simulink model "MissionSupervisor"  (R2020a)
settings: Solver=VariableStepAuto  StartTime=0.0  StopTime=10.0  RelTol=1e-3
undefined symbols (not defined in the file or in its folder): DiscIntNeverNeededParam
libraries: simulink x2
(part 1 of 2)
settings Model: PauseTimes=1  PacingRate=0.350000  Creator=User  LastModifiedBy=User

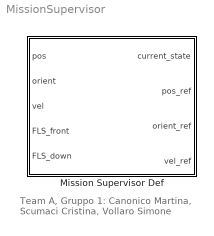
== system MissionSupervisor ==
  note: Team A, Gruppo 1:
      | Canonico Martina, Scumaci Cristina, Vollaro Simone
  Mission Supervisor Def : Subsystem

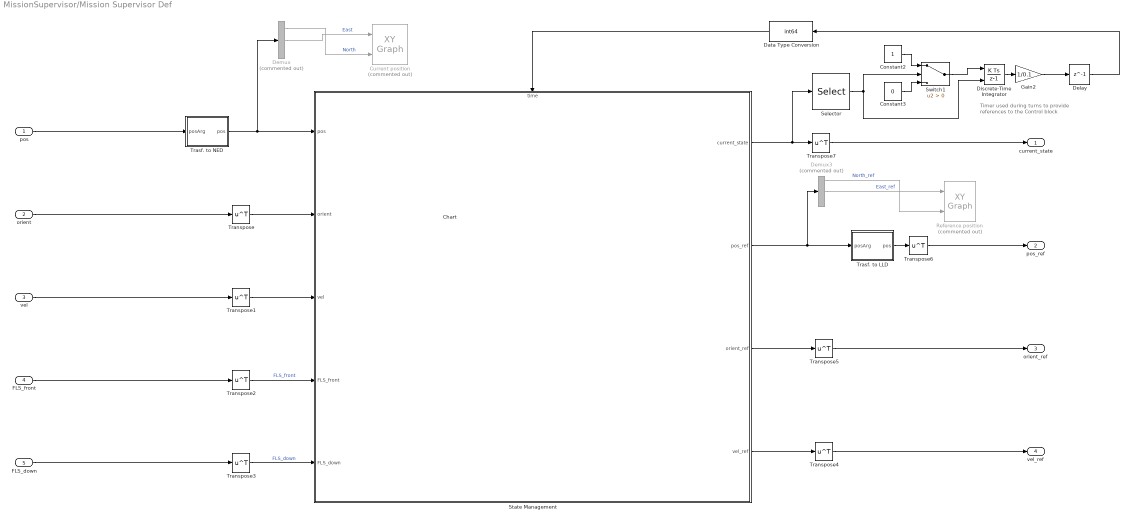
== system MissionSupervisor/Mission Supervisor Def ==
  note: Timer used during turns to
      | provide references to the Control block
  pos : Inport
  orient : Inport  Port=2  PortDimensions=[3 1]
  vel : Inport  Port=3  PortDimensions=[6 1]
  FLS_front : Inport  Port=4  PortDimensions=1
  FLS_down : Inport  Port=5  PortDimensions=1
  Chart : Stateflow chart  TreatAsAtomicUnit=on
  Constant2 : Constant
  Constant3 : Constant  Value=0
  Current position : simulink/Sinks/XY Graph  Commented=on  xmin=0  xmax=150  ymin=0  ymax=150  st=-1
  Data Type Conversion : DataTypeConversion  OutDataTypeStr=int64
  Delay : Delay  DelayLength=1  SampleTime=0.1
  Demux : Demux  Commented=on  Outputs=3
  Demux3 : Demux  Commented=on  Outputs=3
  Discrete-Time Integrator : DiscreteIntegrator  ExternalReset=falling  SampleTime=0.1  ICPrevOutput=DiscIntNeverNeededParam  ICPrevScaledInput=DiscIntNeverNeededParam
  Gain2 : Gain  Gain=1/0.1
  Reference position : simulink/Sinks/XY Graph  Commented=on  xmin=0  xmax=150  ymin=0  ymax=150  st=-1
  Selector : Selector  InputPortWidth=8  IndexOptions=Index vector (dialog)  Indices=4  OutputSizes=1
  State Management : Stateflow chart  TreatAsAtomicUnit=on
      settings: PortSchema="{\"entries\":[{\"content\":{\"sides\":[{\"content\":{\"connectorIds\":[\"In1\",\"In2\",\"In3\",\"In4\",\"In5\"]},\"type\":\"ConnectorPlacement.EquallySpacedRectSide\",\"uuid\":\"b4d768e0-b402-4324-9a12-614211dc6b85\"},{\"content\":{\"connectorIds\":[\"Out1\",\"Out2\",\"Out3\",\"Out4\"],\"side\":\"RIGHT\"},\"type\":\"ConnectorPlacement.EquallySpacedRectSide\",\"uuid\":\"64a4c54a-28a4-456f-aa67-ad7da5d6855f\"},{\"content\":{\"connectorIds\":[\"In6\"],\"side\":\"TOP\"},\"type\":\"ConnectorPlacement.EquallySpacedRectSide\",\"uuid\":\"aacc81fd-f61d-4535-bc25-c566f9f9b0ba\"}]},\"type\":\"ConnectorPlacement.EquallySpacedConnector\",\"uuid\":\"1d5bfe1d-6e45-4fc8-afd6-fe82ea6d1d45\"}],\"packageUris\":[\"http://schema.mathworks.com/mf0/Connector/19700101\"],\"version\":\"1.0\"}"
  Switch1 : Switch  Criteria=u2 > Threshold
  Transpose{,1..7} (8 alike) : Math  Operator=transpose  SaturateOnIntegerOverflow=on
  Trasf. to LLD : MATLAB Function  TreatAsAtomicUnit=on
  Trasf. to NED : MATLAB Function  TreatAsAtomicUnit=on
  current_state : Outport
  pos_ref : Outport  Port=2
  orient_ref : Outport  Port=3
  vel_ref : Outport  Port=4  PortDimensions=[6 1]
  wires:
  Transpose3/1 -> State Management/5(FLS_down)  "FLS_down"
  FLS_front/1 -> Transpose2/1
  Transpose5/1 -> orient_ref/1
  orient/1 -> Transpose/1
  vel/1 -> Transpose1/1
  Transpose4/1 -> vel_ref/1
  FLS_down/1 -> Transpose3/1
  Demux/1 -> Current position/2  "North"
  Demux/2 -> Current position/1  "East"
  Transpose/1 -> State Management/2(orient)
  Transpose1/1 -> State Management/3(vel)
  Transpose2/1 -> State Management/4(FLS_front)  "FLS_front"
  Demux3/1 -> Reference position/2  "North_ref"
  Demux3/2 -> Reference position/1  "East_ref"
  State Management/3(orient_ref) -> Transpose5/1
  State Management/4(vel_ref) -> Transpose4/1
  pos/1 -> Trasf. to NED/1(posArg)
  State Management/2(pos_ref) -> Trasf. to LLD/1(posArg), Demux3/1
  Trasf. to LLD/1(pos) -> Transpose6/1
  Trasf. to NED/1(pos) -> Demux/1, State Management/1(pos)
  Transpose6/1 -> pos_ref/1
  Transpose7/1 -> current_state/1
  Discrete-Time Integrator/1 -> Gain2/1
  Selector/1 -> Discrete-Time Integrator/2, Switch1/2
  Switch1/1 -> Discrete-Time Integrator/1
  Constant3/1 -> Switch1/3
  Constant2/1 -> Switch1/1
  Data Type Conversion/1 -> State Management/6(time)
  Gain2/1 -> Delay/1
  Delay/1 -> Data Type Conversion/1
  State Management/1(current_state) -> Selector/1, Transpose7/1

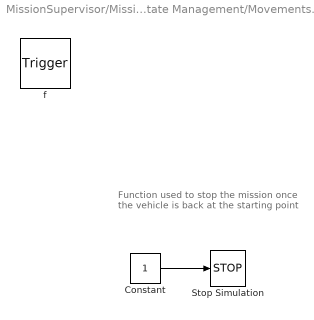
== system MissionSupervisor/Mission Supervisor Def/State Management/Movements.End ==
  note: Function used to stop the mission once
      | the vehicle is back at the starting point
  f : TriggerPort  TriggerType=function-call  VariantControl=(inherit)
      settings: CopyFcn=Stateflow.SLINSF.SimulinkMan.removeBlockPreDeleteFcn  PreDeleteFcn=Stateflow.SLINSF.SimulinkMan.unsafePredeleteFcn
  Constant : Constant
  Stop Simulation : Stop
  wires:
  Constant/1 -> Stop Simulation/1

== matlab function MissionSupervisor/Mission Supervisor Def/Trasf. to NED ==
  data: posArg input; pos output; areaOfInterestCorner parameter
function pos = LLD2NED(posArg,areaOfInterestCorner)
    coder.extrinsic('evalin','wgs84Ellipsoid','geodetic2ned');
    pos = zeros(1,3);
    pos1 = 0;
    pos2 = 0;
    pos3 = 0;
    [pos1, pos2, pos3] = geodetic2ned(posArg(1), posArg(2), posArg(3),areaOfInterestCorner(1), areaOfInterestCorner(2), 0,wgs84Ellipsoid);
    pos = [pos1, pos2, posArg(3)];
end

== matlab function MissionSupervisor/Mission Supervisor Def/Trasf. to LLD ==
  data: posArg input; pos output; areaOfInterestCorner parameter
function pos = NED2LLD(posArg,areaOfInterestCorner)
    coder.extrinsic('evalin','wgs84Ellipsoid','ned2geodetic');
    pos = zeros(1,3);
    pos1 = 0;
    pos2 = 0;
    pos3 = 0;
    [pos1, pos2, pos3] = ned2geodetic(posArg(1), posArg(2), posArg(3),areaOfInterestCorner(1), areaOfInterestCorner(2), 0,wgs84Ellipsoid);
    pos = [pos1, pos2, posArg(3)];%-posArg(3)];
end

== stateflow chart MissionSupervisor/Mission Supervisor Def/Chart ==
